simulink model "SimPIDlong2020b"  (R2021b)
settings: Solver=VariableStepAuto  StartTime=0.0  StopTime=10  RelTol=1e-3
values from neighbouring files (symbols this model uses):
  g_q = tf(modelo(3,1))    [longPID.m]
  Kd = 1.5    [longPID.m]
  Ki = 2    [longPID.m]
  Kp = 4.7    [longPID.m]
libraries: simulink x2, slpidlib x2
settings Model: Creator=danie  LastModifiedBy=Daniel
settings SolverCC: AlgebraicLoopSolver=TrustRegion
settings DebuggingCC: UnconnectedInputMsg=none  UnconnectedOutputMsg=none  UnconnectedLineMsg=none

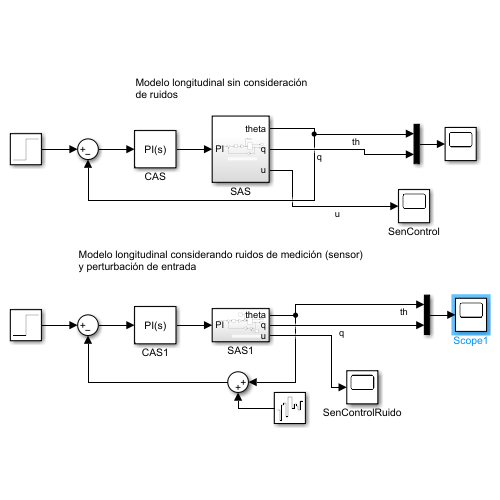
[thumbnail: Simulink's stored preview of the top-level diagram]
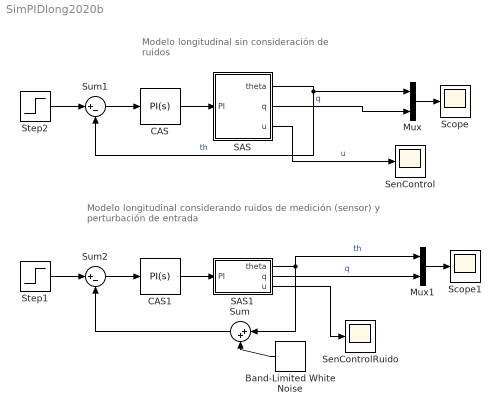
== system SimPIDlong2020b ==
  note: Modelo longitudinal considerando ruidos de medición (sensor)
      | y perturbación de entrada
  note: Modelo longitudinal sin consideración
      | de ruidos
  Band-Limited White Noise : simulink/Sources/Band-Limited White Noise  Cov=[0.0001]  Ts=0.1  seed=[23341]
  CAS : slpidlib/PID Controller  Controller=PI  Form=Parallel  TimeDomain=Continuous-time  UseExternalTs=off  SampleTime=-1  IntegratorMethod=Forward Euler  FilterMethod=Forward Euler  ControllerParametersSource=internal  P=Kp  I=Ki  D=0  UseFilter=on  N=100  TunerSelectOption=Transfer Function Based (PID Tuner App)  InitialConditionSource=internal  InitialConditionForIntegrator=0  InitialConditionForFilter=0  DifferentiatorICPrevScaledInput=0  ExternalReset=none  TrackingMode=off  Kt=1  LimitOutput=off  SatLimitsSource=internal  UpperSaturationLimit=inf  LowerSaturationLimit=-inf  LinearizeAsGain=on  AntiWindupMode=none  Kb=1  POutMin=[]  POutMax=[]  IOutMin=[]  IOutMax=[]  DOutMin=[]  DOutMax=[]  NOutMin=[]  NOutMax=[]  SumOutMin=[]  SumOutMax=[]  SaturationOutMin=[]  SaturationOutMax=[]  PParamMin=[]  PParamMax=[]  IParamMin=[]  IParamMax=[]  DParamMin=[]  DParamMax=[]  NParamMin=[]  NParamMax=[]  KbParamMin=[]  KbParamMax=[]  KtParamMin=[]  KtParamMax=[]  KbOutMin=[]  KbOutMax=[]  KtOutMin=[]  KtOutMax=[]  IntegratorOutMin=[]  IntegratorOutMax=[]  FilterOutMin=[]  FilterOutMax=[]  SumI1OutMin=[]  SumI1OutMax=[]  SumI2OutMin=[]  SumI2OutMax=[]  SumI3OutMin=[]  SumI3OutMax=[]  SumI4OutMin=[]  SumI4OutMax=[]  SumDOutMin=[]  SumDOutMax=[]  DifferentiatorOutMin=[]  DifferentiatorOutMax=[]  FilterDiffOutCoefMin=[]  FilterDiffOutCoefMax=[]  ReciprocalOutMin=[]  ReciprocalOutMax=[]  SumDenOutMin=[]  SumDenOutMax=[]  SumNumOutMin=[]  SumNumOutMax=[]  DivideOutMin=[]  DivideOutMax=[]  UdiffTsProdOutMin=[]  UdiffTsProdOutMax=[]  NTsProdOutMin=[]  NTsProdOutMax=[]  UintegralTsProdOutMin=[]  UintegralTsProdOutMax=[]  UngainTsProdOutMin=[]  UngainTsProdOutMax=[]  IntegratorContinuousStateAttributes=''  IntegratorStateMustResolveToSignalObject=off  IntegratorRTWStateStorageClass=Auto  FilterContinuousStateAttributes=''  FilterStateMustResolveToSignalObject=off  FilterRTWStateStorageClass=Auto  ParallelPVariant=InternalParameters  IdealPVariant=Disabled  IVariant=InternalParameters  DVariant=Disabled  IntegratorVariant=Continuous  SatVariant=Disabled  AWVariant=Passthrough  PCopyVariant=Disabled  TRVariant=Disabled  FdbkBlocksVariant=Forward  IdealPFdbkVariant=Disabled  SatFdbkVariant=Disabled  DerivativeFilterVariant=Disabled  NVariant=Disabled  NCopyVariant=Disabled_SignalSpec  FilterICVariant=Disabled  IntegratorICVariant=InternalICs  ExternalResetVariant=Disabled  TRSumVariant=Passthrough  SumFdbkVariant=Disabled  SumVariant=Sum_PI  TsampFilterVariant=InternalTs  TsampNgainVariant=Passthrough  TsampIntegralVariant=Passthrough  ExternalSaturationOutDataTypeStr=Inherit: Same as second input
  CAS1 : slpidlib/PID Controller  Controller=PI  Form=Parallel  TimeDomain=Continuous-time  UseExternalTs=off  SampleTime=-1  IntegratorMethod=Forward Euler  FilterMethod=Forward Euler  ControllerParametersSource=internal  P=Kp  I=Ki  D=0  UseFilter=on  N=100  TunerSelectOption=Transfer Function Based (PID Tuner App)  InitialConditionSource=internal  InitialConditionForIntegrator=0  InitialConditionForFilter=0  DifferentiatorICPrevScaledInput=0  ExternalReset=none  TrackingMode=off  Kt=1  LimitOutput=off  SatLimitsSource=internal  UpperSaturationLimit=inf  LowerSaturationLimit=-inf  LinearizeAsGain=on  AntiWindupMode=none  Kb=1  POutMin=[]  POutMax=[]  IOutMin=[]  IOutMax=[]  DOutMin=[]  DOutMax=[]  NOutMin=[]  NOutMax=[]  SumOutMin=[]  SumOutMax=[]  SaturationOutMin=[]  SaturationOutMax=[]  PParamMin=[]  PParamMax=[]  IParamMin=[]  IParamMax=[]  DParamMin=[]  DParamMax=[]  NParamMin=[]  NParamMax=[]  KbParamMin=[]  KbParamMax=[]  KtParamMin=[]  KtParamMax=[]  KbOutMin=[]  KbOutMax=[]  KtOutMin=[]  KtOutMax=[]  IntegratorOutMin=[]  IntegratorOutMax=[]  FilterOutMin=[]  FilterOutMax=[]  SumI1OutMin=[]  SumI1OutMax=[]  SumI2OutMin=[]  SumI2OutMax=[]  SumI3OutMin=[]  SumI3OutMax=[]  SumI4OutMin=[]  SumI4OutMax=[]  SumDOutMin=[]  SumDOutMax=[]  DifferentiatorOutMin=[]  DifferentiatorOutMax=[]  FilterDiffOutCoefMin=[]  FilterDiffOutCoefMax=[]  ReciprocalOutMin=[]  ReciprocalOutMax=[]  SumDenOutMin=[]  SumDenOutMax=[]  SumNumOutMin=[]  SumNumOutMax=[]  DivideOutMin=[]  DivideOutMax=[]  UdiffTsProdOutMin=[]  UdiffTsProdOutMax=[]  NTsProdOutMin=[]  NTsProdOutMax=[]  UintegralTsProdOutMin=[]  UintegralTsProdOutMax=[]  UngainTsProdOutMin=[]  UngainTsProdOutMax=[]  IntegratorContinuousStateAttributes=''  IntegratorStateMustResolveToSignalObject=off  IntegratorRTWStateStorageClass=Auto  FilterContinuousStateAttributes=''  FilterStateMustResolveToSignalObject=off  FilterRTWStateStorageClass=Auto  ParallelPVariant=InternalParameters  IdealPVariant=Disabled  IVariant=InternalParameters  DVariant=Disabled  IntegratorVariant=Continuous  SatVariant=Disabled  AWVariant=Passthrough  PCopyVariant=Disabled  TRVariant=Disabled  FdbkBlocksVariant=Forward  IdealPFdbkVariant=Disabled  SatFdbkVariant=Disabled  DerivativeFilterVariant=Disabled  NVariant=Disabled  NCopyVariant=Disabled_SignalSpec  FilterICVariant=Disabled  IntegratorICVariant=InternalICs  ExternalResetVariant=Disabled  TRSumVariant=Passthrough  SumFdbkVariant=Disabled  SumVariant=Sum_PI  TsampFilterVariant=InternalTs  TsampNgainVariant=Passthrough  TsampIntegralVariant=Passthrough  ExternalSaturationOutDataTypeStr=Inherit: Same as second input
  Mux : Mux  Inputs=2
  Mux1 : Mux  Inputs=2
  SAS : Subsystem
  SAS1 : Subsystem
  Scope : Scope
  Scope1 : Scope
  SenControl : Scope
  SenControlRuido : Scope
  Step1 : Step  After=40  SampleTime=0
  Step2 : Step  After=40  SampleTime=0
  Sum : Sum  Inputs=|++
  Sum1 : Sum  Inputs=|+-
  Sum2 : Sum  Inputs=|+-
  wires:
  Sum1/1 -> CAS/1
  SAS/1(theta) -> Mux/1, Sum1/2  "th"
  SAS/2(q) -> Mux/2  "q"
  CAS/1 -> SAS/1(PI)
  Step2/1 -> Sum1/1
  Step1/1 -> Sum2/1
  CAS1/1 -> SAS1/1(PI)
  SAS1/2(q) -> Mux1/2  "q"
  SAS1/1(theta) -> Mux1/1, Sum/1  "th"
  Sum2/1 -> CAS1/1
  Band-Limited White Noise/1 -> Sum/2
  Sum/1 -> Sum2/2
  SAS/3(u) -> SenControl/1  "u"
  SAS1/3(u) -> SenControlRuido/1
  Mux/1 -> Scope/1
  Mux1/1 -> Scope1/1

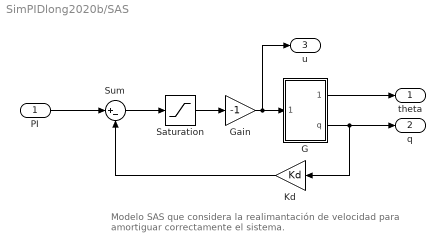
== system SimPIDlong2020b/SAS ==
  note: Modelo SAS que considera la realimantación de velocidad
      | para amortiguar correctamente el sistema.
  PI : Inport
  G : Subsystem
  Gain : Gain  Gain=-1
  Kd : Gain  Gain=Kd
  Saturation : Saturate  UpperLimit=30  LowerLimit=-30
  Sum : Sum  Inputs=|+-
  theta : Outport
  q : Outport  Port=2
  u : Outport  Port=3
  wires:
  G/2(q) -> q/1, Kd/1
  Kd/1 -> Sum/2
  G/1(theta) -> theta/1
  PI/1 -> Sum/1
  Sum/1 -> Saturation/1
  Gain/1 -> u/1, G/1(Elev)
  Saturation/1 -> Gain/1

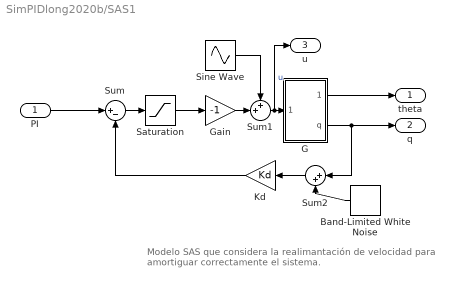
== system SimPIDlong2020b/SAS1 ==
  note: Modelo SAS que considera la realimantación de velocidad
      | para amortiguar correctamente el sistema.
  PI : Inport
  Band-Limited White Noise : simulink/Sources/Band-Limited White Noise  Cov=[0.0001]  Ts=0.1  seed=[23341]
  G : Subsystem
  Gain : Gain  Gain=-1
  Kd : Gain  Gain=Kd
  Saturation : Saturate  UpperLimit=30  LowerLimit=-30
  Sine Wave : Sin  Frequency=12*pi  SampleTime=0
  Sum : Sum  Inputs=|+-
  Sum1 : Sum  Inputs=++|
  Sum2 : Sum  Inputs=|++
  theta : Outport
  q : Outport  Port=2
  u : Outport  Port=3
  wires:
  Saturation/1 -> Gain/1
  Sum/1 -> Saturation/1
  PI/1 -> Sum/1
  G/1(theta) -> theta/1
  Kd/1 -> Sum/2
  G/2(q) -> Sum2/1, q/1
  Gain/1 -> Sum1/2
  Sum1/1 -> u/1, G/1(Elev)  "u"
  Sine Wave/1 -> Sum1/1
  Sum2/1 -> Kd/1
  Band-Limited White Noise/1 -> Sum2/2

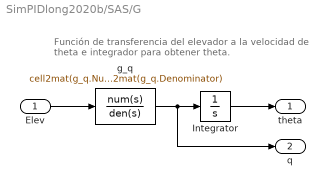
== system SimPIDlong2020b/SAS/G ==
  note: Función de transferencia del elevador a la velocidad
      | de theta e integrador para obtener theta.
  Elev : Inport
  Integrator : Integrator
  g_q : TransferFcn  Numerator=cell2mat(g_q.Numerator)  Denominator=cell2mat(g_q.Denominator)
  theta : Outport
  q : Outport  Port=2
  wires:
  Elev/1 -> g_q/1
  g_q/1 -> q/1, Integrator/1
  Integrator/1 -> theta/1

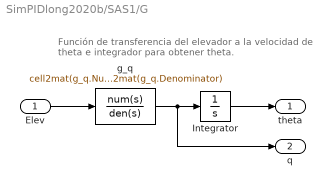
== system SimPIDlong2020b/SAS1/G ==
  note: Función de transferencia del elevador a la velocidad
      | de theta e integrador para obtener theta.
  Elev : Inport
  Integrator : Integrator
  g_q : TransferFcn  Numerator=cell2mat(g_q.Numerator)  Denominator=cell2mat(g_q.Denominator)
  theta : Outport
  q : Outport  Port=2
  wires:
  Integrator/1 -> theta/1
  g_q/1 -> Integrator/1, q/1
  Elev/1 -> g_q/1
